simulink library "FCM_lib"  (Simulink 7.4)
settings: Solver=ode45  StartTime=0.0  StopTime=10.0  RelTol=1e-3
values from neighbouring files (symbols this model uses):
  FCMc_c_BCPNomEngy = mpt.Parameter    [FCM_CAL.m]
  FCMc_c_BRMRatCpty = mpt.Parameter    [FCM_CAL.m]
  FCMc_enum_BRMBattType = mpt.Parameter    [FCM_CAL.m]
  FCMc_i_ConstCurReq = mpt.Parameter    [FCM_CAL.m]
  FCMc_i_CurDifThrld = mpt.Parameter    [FCM_CAL.m]
  FCMc_i_CurReq_min = mpt.Parameter    [FCM_CAL.m]
  FCMc_num_BRMProtolVer = mpt.Parameter    [FCM_CAL.m]
  FCMc_t_CellTemp_MaxAlwd = mpt.Parameter    [FCM_CAL.m]
  FCMc_t_CellTemp_MinAlwd = mpt.Parameter    [FCM_CAL.m]
  FCMc_tm_ConstVoltTime = mpt.Parameter    [FCM_CAL.m]
  FCMc_tm_FastEndCondt = mpt.Parameter    [FCM_CAL.m]
  FCMc_v_BRMPackRatVolt = mpt.Parameter    [FCM_CAL.m]
  FCMc_v_VoltDifThrld = mpt.Parameter    [FCM_CAL.m]
  FCMm_c_CellChaC_AH = mpt.Parameter    [FCM_CAL.m]
  FCMm_i_CurrArrayT = mpt.Parameter    [FCM_CAL.m]
  FCMx_t_CelltempArrayT = mpt.Parameter    [FCM_CAL.m]
undefined symbols (not defined in the file or in its folder): BATc_pct_PackSocAlwd, BATc_v_CellVolt_MaxAlwd, BATc_v_CellVolt_MinAlwd, BATc_v_ConstVoltCell, BATc_v_PackVoltAlwd, FCM_Charging_St, PACK_Const_ParaCellNumOfMdl
libraries: Defined_Functionality x18
(part 1 of 2)
settings Model: Creator=sunsijun  LastModifiedBy=sunsijun

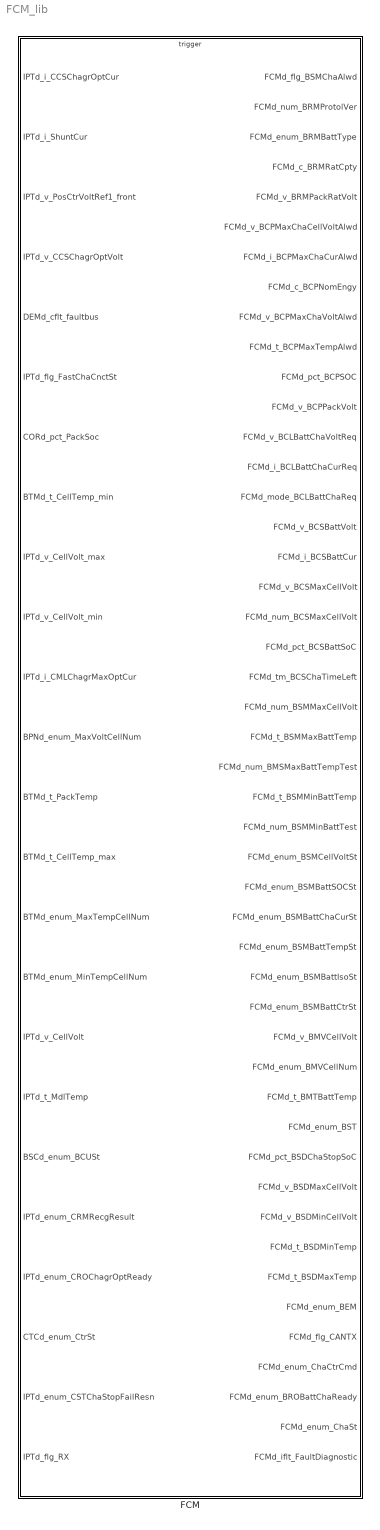
== system FCM_lib ==
  FCM : Subsystem  Description=|  TreatAsAtomicUnit=on
      | $Author:zwy
      | $Date:2015/05/12$    
      | $Revision:1.0$
      settings: RTWSystemCode=Function  RTWFcnNameOpts=Use subsystem name

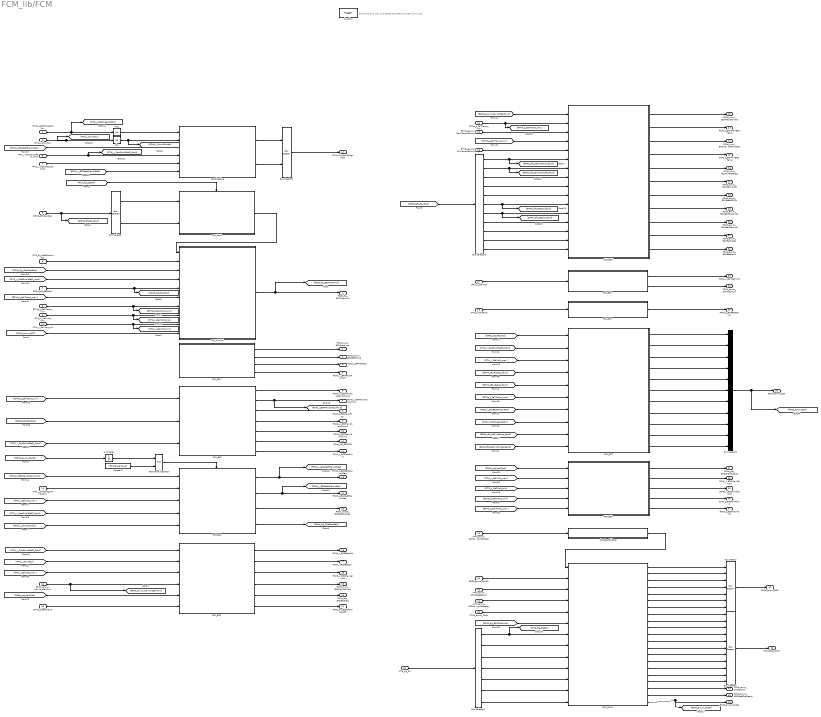
== system FCM_lib/FCM ==
  note: $Author:Zhang Weiyou$
      | $Date:2015/06/10-$
      | $Revision:1.0$
  IPTd_i_CCSChagrOptCur : Inport
  IPTd_i_ShuntCur : Inport  Port=2
  IPTd_v_PosCtrVoltRef1_front : Inport  Port=3
  IPTd_v_CCSChagrOptVolt : Inport  Port=4
  DEMd_cflt_faultbus : Inport  Port=5
  IPTd_flg_FastChaCnctSt : Inport  Port=6
  CORd_pct_PackSoc : Inport  Port=7
  BTMd_t_CellTemp_min : Inport  Port=8
  IPTd_v_CellVolt_max : Inport  Port=9
  IPTd_v_CellVolt_min : Inport  Port=10
  IPTd_i_CMLChagrMaxOptCur : Inport  Port=11
  BPNd_enum_MaxVoltCellNum : Inport  Port=12
  BTMd_t_PackTemp : Inport  Port=13
  BTMd_t_CellTemp_max : Inport  Port=14
  BTMd_enum_MaxTempCellNum : Inport  Port=15
  BTMd_enum_MinTempCellNum : Inport  Port=16
  IPTd_v_CellVolt : Inport  Port=17
  IPTd_t_MdlTemp : Inport  Port=18
  BSCd_enum_BCUSt : Inport  Port=19
  IPTd_enum_CRMRecgResult : Inport  Port=20
  IPTd_enum_CROChagrOptReady : Inport  Port=21
  CTCd_enum_CtrSt : Inport  Port=22
  IPTd_enum_CSTChaStopFailResn : Inport  Port=23
  IPTd_flg_RX : Inport  Port=24
  function : TriggerPort  TriggerType=function-call
  Abs : Abs
  Abs1 : Abs
  Bus Creator : BusCreator  Inputs=7
  Bus Creator1 : BusCreator  Inputs=11
  Bus Creator2 : BusCreator  Inputs=11
  Bus Creator3 : BusCreator  Inputs=2
  Bus Selector : BusSelector  OutputSignals=FCM_Fault_Bus.FCMd_cflt_ChaCurDifOver_faultRaw,FCM_Fault_Bus.FCMd_cflt_ChaVoltDifOver_faultRaw
  Bus Selector1 : BusSelector  OutputSignals=BPN_Fault_Bus.BPNd_cflt_CellVoltOver_faultRaw,BPN_Fault_Bus.BPNd_cflt_CellVoltUnder_faultRaw,BPN_Fault_Bus.BPNd_cflt_PackVoltUnder_faultRaw,BPN_Fault_Bus.BPNd_cflt_PackVoltOver_faultRaw,BPN_Fault_Bus.BPNd_cflt_ChaCurOver_faultRaw,EHP_Fault_Bus.EHPd_cflt_PosIso_faultRaw,EHP_Fault_Bus.EHPd_cflt_NegIso_faultRaw,CTC_Fault_Bus.CTCd_cflt_PosCtrStuckOpen_faultRaw,CTC_Fault_Bus.CTCd_cflt_PosCtrStuckCld_faultRaw,CTC_Fault_Bus.CTCd_cflt_NegCtrStuckOpen_faultRaw,CTC_Fault_Bus.CTCd_cflt_NegCtrStuckCld_faultRaw
  Bus Selector2 : BusSelector  OutputSignals=IPTd_flg_CCSRX,IPTd_flg_CMLRX,IPTd_flg_CRORX,IPTd_flg_CSDRX,IPTd_flg_CSTRX,IPTd_flg_CTSRX,IPTd_flg_CRMRX
  ChaStopFailResn : Subsystem
  Constant : Constant  Value=FCM_Charging_St  OutDataTypeMode=uint8  OutDataType=fixdt(1, 16)  OutScaling=2^0  OutDataTypeStr=uint8
  FCM_BCL : Subsystem
      settings: RTWFcnNameOpts=Use subsystem name  RTWFileNameOpts=Use subsystem name
  FCM_BCP : Subsystem
      settings: RTWFcnNameOpts=Use subsystem name  RTWFileNameOpts=Use subsystem name
  FCM_BCS : Subsystem
      settings: RTWFcnNameOpts=Use subsystem name  RTWFileNameOpts=Use subsystem name
  FCM_BMT : Subsystem
      settings: RTWFcnNameOpts=Use subsystem name  RTWFileNameOpts=Use subsystem name
  FCM_BMV : Subsystem
      settings: RTWFcnNameOpts=Use subsystem name  RTWFileNameOpts=Use subsystem name
  FCM_BRM : Subsystem
      settings: RTWFcnNameOpts=Use subsystem name  RTWFileNameOpts=Use subsystem name
  FCM_BSD : Subsystem
      settings: RTWFcnNameOpts=Use subsystem name  RTWFileNameOpts=Use subsystem name
  FCM_BSM : Subsystem
      settings: RTWFcnNameOpts=Use subsystem name  RTWFileNameOpts=Use subsystem name
  FCM_BST : Subsystem
      settings: RTWFcnNameOpts=Use subsystem name  RTWFileNameOpts=Use subsystem name
  FCM_ChAlwd : Subsystem
      settings: RTWFcnNameOpts=Use subsystem name  RTWFileNameOpts=Use subsystem name
  FCM_FLOW : Stateflow chart
      settings: RTWFcnNameOpts=Use subsystem name  RTWFileNameOpts=Use subsystem name
  FCM_fault : Subsystem  Description=|
      | $Author:Zhao XiangRi$
      | $Date:2015/03/30$    
      | $Revision:1.0$
  FastChaDiag : Subsystem  Description=|
      | $Author:Zhao XiangRi$
      | $Date:2015/03/30$    
      | $Revision:1.0$
  Relational Operator : RelationalOperator  Operator===  LogicOutDataTypeMode=boolean  LogicDataType=fixdt(0, 8)  OutDataTypeStr=boolean
  Unit Delay : UnitDelay  SampleTime=-1
  FCMd_flg_BSMChaAlwd : Outport
  FCMd_num_BRMProtolVer : Outport  Port=2
  FCMd_enum_BRMBattType : Outport  Port=3
  FCMd_c_BRMRatCpty : Outport  Port=4
  FCMd_v_BRMPackRatVolt : Outport  Port=5
  FCMd_v_BCPMaxChaCellVoltAlwd : Outport  Port=6
  FCMd_i_BCPMaxChaCurAlwd : Outport  Port=7
  FCMd_c_BCPNomEngy : Outport  Port=8
  FCMd_v_BCPMaxChaVoltAlwd : Outport  Port=9
  FCMd_t_BCPMaxTempAlwd : Outport  Port=10
  FCMd_pct_BCPSOC : Outport  Port=11
  FCMd_v_BCPPackVolt : Outport  Port=12
  FCMd_v_BCLBattChaVoltReq : Outport  Port=13
  FCMd_i_BCLBattChaCurReq : Outport  Port=14
  FCMd_mode_BCLBattChaReq : Outport  Port=15
  FCMd_v_BCSBattVolt : Outport  Port=16
  FCMd_i_BCSBattCur : Outport  Port=17
  FCMd_v_BCSMaxCellVolt : Outport  Port=18
  FCMd_num_BCSMaxCellVolt : Outport  Port=19
  FCMd_pct_BCSBattSoC : Outport  Port=20
  FCMd_tm_BCSChaTimeLeft : Outport  Port=21
  FCMd_num_BSMMaxCellVolt : Outport  Port=22
  FCMd_t_BSMMaxBattTemp : Outport  Port=23
  FCMd_num_BMSMaxBattTempTest : Outport  Port=24
  FCMd_t_BSMMinBattTemp : Outport  Port=25
  FCMd_num_BSMMinBattTest : Outport  Port=26
  FCMd_enum_BSMCellVoltSt : Outport  Port=27
  FCMd_enum_BSMBattSOCSt : Outport  Port=28
  FCMd_enum_BSMBattChaCurSt : Outport  Port=29
  FCMd_enum_BSMBattTempSt : Outport  Port=30
  FCMd_enum_BSMBattIsoSt : Outport  Port=31
  FCMd_enum_BSMBattCtrSt : Outport  Port=32
  FCMd_v_BMVCellVolt : Outport  Port=33
  FCMd_enum_BMVCellNum : Outport  Port=34  InitialOutput=0
  FCMd_t_BMTBattTemp : Outport  Port=35
  FCMd_enum_BST : Outport  Port=36
  FCMd_pct_BSDChaStopSoC : Outport  Port=37
  FCMd_v_BSDMaxCellVolt : Outport  Port=38
  FCMd_v_BSDMinCellVolt : Outport  Port=39
  FCMd_t_BSDMinTemp : Outport  Port=40
  FCMd_t_BSDMaxTemp : Outport  Port=41
  FCMd_enum_BEM : Outport  Port=42
  FCMd_flg_CANTX : Outport  Port=43
  FCMd_enum_ChaCtrCmd : Outport  Port=44
  FCMd_enum_BROBattChaReady : Outport  Port=45
  FCMd_enum_ChaSt : Outport  Port=46
  FCMd_iflt_FaultDiagnostic : Outport  Port=47
  wires:
  Relational Operator/1 -> FCM_BCL/Enable
  Unit Delay/1 -> Relational Operator/1
  Constant/1 -> Relational Operator/2
  [FCMd_enum_ChaSt] -> Unit Delay/1
  [IPTd_flg_CCSRX] -> FCM_fault/Enable
  [FCMd_enum_BST] -> FCM_ChAlwd/10(FCMd_enum_BST)
  FCM_fault/1(FCMd_flg_fault) -> FCM_ChAlwd/1(FCMd_flg_fault)
  Abs/1 -> [FCMd_i_ShuntCurAbs], FastChaDiag/2(FCMd_i_ShuntCurAbs)  "FCMd_i_ShuntCurAbs"
  Abs1/1 -> FastChaDiag/1(FCMd_i_CCSChagrOptCurAbs)  "FCMd_i_CCSChagrOptCurAbs"
  [IPTd_v_PosCtrVoltRef1_front] -> FCM_ChAlwd/4(IPTd_v_PosCtrVoltRef1_front)
  DEMd_cflt_faultbus/1 -> [DEMd_cflt_faultbus], Bus Selector/1
  Bus Creator3/1 -> FCMd_iflt_FaultDiagnostic/1  "FCMd_iflt_FaultDiagnostic"
  FastChaDiag/2(FCMd_iflt_ChaVoltDifOver_fault) -> Bus Creator3/2
  FastChaDiag/1(FCMd_iflt_ChaCurDifOver_fault) -> Bus Creator3/1
  [FCMd_v_BCLBattChaVoltReq] -> FastChaDiag/6(FCMd_v_BCLBattChaVoltReq)
  IPTd_v_CCSChagrOptVolt/1 -> FastChaDiag/5(IPTd_v_CCSChagrOptVolt)
  [FCMd_i_BCLBattChaCurReq] -> FastChaDiag/3(FCMd_i_BCLBattChaCurReq)
  IPTd_v_PosCtrVoltRef1_front/1 -> [IPTd_v_PosCtrVoltRef1_front], FastChaDiag/4(IPTd_v_PosCtrVoltRef1_front)
  IPTd_i_CCSChagrOptCur/1 -> [IPTd_i_CCSChagrOptCur], Abs1/1
  [FCMd_i_ShuntCurAbs] -> FCM_BCL/5(FCMd_i_ShuntCurAbs)
  Bus Selector2/7 -> FCM_FLOW/13(IPTd_flg_CRMRX)  "<IPTd_flg_CRMRX>"
  Bus Selector2/2 -> FCM_FLOW/8(IPTd_flg_CMLRX)  "<IPTd_flg_CMLRX>"
  Bus Selector2/6 -> FCM_FLOW/12(IPTd_flg_CTSRX)  "<IPTd_flg_CTSRX>"
  Bus Selector2/1 -> [IPTd_flg_CCSRX], FCM_FLOW/7(IPTd_flg_CCSRX)  "<IPTd_flg_CCSRX>"
  Bus Selector2/4 -> FCM_FLOW/10(IPTd_flg_CSDRX)  "<IPTd_flg_CSDRX>"
  Bus Selector2/5 -> FCM_FLOW/11(IPTd_flg_CSTRX)  "<IPTd_flg_CSTRX>"
  Bus Selector2/3 -> FCM_FLOW/9(IPTd_flg_CRORX)  "<IPTd_flg_CRORX>"
  FCM_FLOW/20(FCMd_enum_BROBattChaReady) -> FCMd_enum_BROBattChaReady/1  "FCMd_enum_BROBattChaReady"
  FCM_FLOW/19(FCMd_enum_ChaCtrCmd) -> FCMd_enum_ChaCtrCmd/1  "FCMd_enum_ChaCtrCmd"
  [DEMd_cflt_faultbus] -> Bus Selector1/1
  FCM_BCL/4(FCMd_flg_ChaStopReq) -> [FCMd_flg_ChaStopReq]
  [EHPd_cflt_POSIso_fault] -> FCM_BST/4(EHPd_cflt_POSIso_fault)
  [EHPd_cflt_NegIso_fault] -> FCM_BST/5(EHPd_cflt_NegIso_fault)
  [BTMd_t_CellTemp_max] -> FCM_BST/6(BTMd_t_CellTemp_max)
  [CORd_pct_PackSoc] -> FCM_BSD/1(CORd_pct_PackSoc)
  [BTMd_t_CellTemp_max] -> FCM_BSD/5(BTMd_t_CellTemp_max)
  [BTMd_t_CellTemp_min] -> FCM_BSD/4(BTMd_t_CellTemp_min)
  FCM_BSD/1(FCMd_pct_BSDChaStopSoC) -> FCMd_pct_BSDChaStopSoC/1
  FCM_BSD/2(FCMd_v_BSDMaxCellVolt) -> FCMd_v_BSDMaxCellVolt/1
  FCM_BSD/3(FCMd_v_BSDMinCellVolt) -> FCMd_v_BSDMinCellVolt/1
  FCM_BSD/4(FCMd_t_BSDMinTemp) -> FCMd_t_BSDMinTemp/1
  FCM_BSD/5(FCMd_t_BSDMaxTemp) -> FCMd_t_BSDMaxTemp/1
  [IPTd_v_CellVolt_max] -> FCM_BSD/2(IPTd_v_CellVolt_max)
  [IPTd_v_CellVolt_min] -> FCM_BSD/3(IPTd_v_CellVolt_min)
  [BPNd_cflt_CellVoltOver_fault] -> FCM_BST/9(BPNd_cflt_CellVoltOver_fault)
  FCM_BST/1(FCMd_enum_BSTChaStopResn1) -> Bus Creator2/1
  FCM_BST/2(FCMd_enum_BSTChaStopResn2) -> Bus Creator2/2
  FCM_BST/3(FCMd_enum_BSTChaStopResn3) -> Bus Creator2/3
  FCM_BST/4(FCMd_enum_BSTChaFailResn1) -> Bus Creator2/4
  FCM_BST/5(FCMd_enum_BSTChaFailResn2) -> Bus Creator2/5
  FCM_BST/6(FCMd_enum_BSTChaFailResn3) -> Bus Creator2/6
  FCM_BST/7(FCMd_enum_BSTChaFailResn4) -> Bus Creator2/7
  FCM_BST/8(FCMd_enum_BSTChaFailResn5) -> Bus Creator2/8
  FCM_BST/9(FCMd_enum_BSTChaFailResn6) -> Bus Creator2/9
  FCM_BST/10(FCMd_enum_BSTChaErrResn1) -> Bus Creator2/10
  FCM_BST/11(FCMd_enum_BSTChaErrResn2) -> Bus Creator2/11
  [CORd_pct_PackSoc] -> FCM_BST/1(CORd_pct_PackSoc)
  [IPTd_v_PosCtrVoltRef1_front] -> FCM_BST/2(IPTd_v_PosCtrVoltRef1_front)
  [IPTd_v_CellVolt_max] -> FCM_BST/3(IPTd_v_CellVolt_max)
  Bus Creator2/1 -> [FCMd_enum_BST], FCMd_enum_BST/1  "FCMd_enum_BST"
  FCM_BCS/1(FCMd_v_BCSBattVolt) -> FCMd_v_BCSBattVolt/1
  FCM_BCS/2(FCMd_i_BCSBattCur) -> FCMd_i_BCSBattCur/1
  FCM_BCS/3(FCMd_v_BCSMaxCellVolt) -> FCMd_v_BCSMaxCellVolt/1
  FCM_BCS/4(FCMd_num_BCSMaxCellVolt) -> FCMd_num_BCSMaxCellVolt/1
  FCM_BCS/5(FCMd_pct_BCSBattSoC) -> FCMd_pct_BCSBattSoC/1
  [IPTd_v_PosCtrVoltRef1_front] -> FCM_BCS/1("IPTd_v_PosCtrVoltRef1_front ")
  BPNd_enum_MaxVoltCellNum/1 -> [BPNd_enum_MaxVoltCellNum], FCM_BCS/4(BPNd_enum_MaxVoltCellNum)
  [IPTd_v_CellVolt_max] -> FCM_BCS/3(IPTd_v_CellVolt_max)
  [CORd_pct_PackSoc] -> FCM_BCS/5(CORd_pct_PackSoc)
  BTMd_t_PackTemp/1 -> FCM_BCS/6(BTMd_t_PackTemp)
  FCM_BCS/6(FCMd_tm_BCSChaTimeLeft) -> FCMd_tm_BCSChaTimeLeft/1
  [IPTd_i_ShuntCur] -> FCM_BCS/2(IPTd_i_ShuntCur)
  Bus Selector1/1 -> FCM_BSM/6(BPNd_cflt_CellVoltOver_fault), [BPNd_cflt_CellVoltOver_fault]  "<BPNd_cflt_CellVoltOver_faultRaw>"
  Bus Selector1/2 -> FCM_BSM/7(BPNd_cflt_CellVoltUnder_fault), [BPNd_cflt_CellVoltUnder_fault]  "<BPNd_cflt_CellVoltUnder_faultRaw>"
  Bus Selector1/3 -> FCM_BSM/8(BPNd_cflt_PackSocUnder_fault)  "<BPNd_cflt_PackVoltUnder_faultRaw>"
  Bus Selector1/4 -> FCM_BSM/9(BPNd_cflt_PackSocOver_fault)  "<BPNd_cflt_PackVoltOver_faultRaw>"
  BTMd_t_CellTemp_max/1 -> FCM_BSM/2(BTMd_t_CellTemp_max), [BTMd_t_CellTemp_max]
  [BPNd_enum_MaxVoltCellNum] -> FCM_BSM/1(BPNd_enum_MaxVoltCellNum)
  BTMd_enum_MaxTempCellNum/1 -> FCM_BSM/3(BTMd_enum_MaxTempCellNum)
  [BTMd_t_CellTemp_min] -> FCM_BSM/4(BTMd_t_CellTemp_min)
  BTMd_enum_MinTempCellNum/1 -> FCM_BSM/5(BTMd_enum_MinTempCellNum)
  Bus Selector1/5 -> FCM_BSM/10(BPNd_cflt_ChaCurOver_fault)  "<BPNd_cflt_ChaCurOver_faultRaw>"
  Bus Selector1/6 -> FCM_BSM/11(EHPd_cflt_POSIso_fault), [EHPd_cflt_POSIso_fault]  "<EHPd_cflt_PosIso_faultRaw>"
  Bus Selector1/7 -> FCM_BSM/12(EHPd_cflt_NegIso_fault), [EHPd_cflt_NegIso_fault]  "<EHPd_cflt_NegIso_faultRaw>"
  Bus Selector1/8 -> FCM_BSM/13(CTCd_cflt_PosCtrStuckOpen_fault)  "<CTCd_cflt_PosCtrStuckOpen_faultRaw>"
  Bus Selector1/9 -> FCM_BSM/14(CTCd_cflt_PosCtrStuckCld_fault)  "<CTCd_cflt_PosCtrStuckCld_faultRaw>"
  Bus Selector1/10 -> FCM_BSM/15(CTCd_cflt_NegCtrtStuckOpen_fault)  "<CTCd_cflt_NegCtrStuckOpen_faultRaw>"
  Bus Selector1/11 -> FCM_BSM/16(CTCd_cflt_NegCtrStuckCld_fault)  "<CTCd_cflt_NegCtrStuckCld_faultRaw>"
  FCM_BSM/6(FCMd_enum_BSMCellVoltSt) -> FCMd_enum_BSMCellVoltSt/1
  FCM_BSM/7(FCMd_enum_BSMBattSOCSt) -> FCMd_enum_BSMBattSOCSt/1
  FCM_BSM/8(FCMd_enum_BSMBattChaCurSt) -> FCMd_enum_BSMBattChaCurSt/1
  FCM_BSM/9(FCMd_enum_BSMBattTempSt) -> FCMd_enum_BSMBattTempSt/1
  FCM_BSM/10(FCMd_enum_BSMBattIsoSt) -> FCMd_enum_BSMBattIsoSt/1
  FCM_BSM/11(FCMd_enum_BSMBattCtrSt) -> FCMd_enum_BSMBattCtrSt/1
  FCM_BSM/1(FCMd_num_BSMMaxCellVolt) -> FCMd_num_BSMMaxCellVolt/1
  FCM_BSM/2(FCMd_t_BSMMaxBattTemp) -> FCMd_t_BSMMaxBattTemp/1
  FCM_BSM/3(FCMd_num_BMSMaxBattTempTest) -> FCMd_num_BMSMaxBattTempTest/1
  FCM_BSM/4(FCMd_t_BSMMinBattTemp) -> FCMd_t_BSMMinBattTemp/1
  FCM_BSM/5(FCMd_num_BSMMinBattTest) -> FCMd_num_BSMMinBattTest/1
  IPTd_i_CMLChagrMaxOptCur/1 -> FCM_BCL/2(IPTd_i_CMLChagrMaxOptCur)
  [FCMd_i_BCPMaxChaCurAlwd] -> FCM_BCL/1(FCMd_i_BCPMaxChaCurAlwd)
  [IPTd_v_PosCtrVoltRef1_front] -> FCM_BCL/4(IPTd_v_PosCtrVoltRef1_front)
  IPTd_i_ShuntCur/1 -> [IPTd_i_ShuntCur], Abs/1
  [IPTd_v_CellVolt_max] -> FCM_BCL/3(IPTd_v_CellVolt_max)
  [IPTd_v_PosCtrVoltRef1_front] -> FCM_BCP/3(IPTd_v_PosCtrVoltRef1_front)
  [CORd_pct_PackSoc] -> FCM_BCP/2(CORd_pct_PackSoc)
  FCM_BCP/7(FCMd_v_BCPPackVolt) -> FCMd_v_BCPPackVolt/1
  FCM_BCP/6(FCMd_pct_BCPSOC) -> FCMd_pct_BCPSOC/1
  FCM_BCP/5(FCMd_t_BCPMaxTempAlwd) -> FCMd_t_BCPMaxTempAlwd/1
  FCM_BCP/3(FCMd_c_BCPNomEngy) -> FCMd_c_BCPNomEngy/1
  [BTMd_t_CellTemp_min] -> FCM_BCP/1(BTMd_t_CellTemp_min)
  FCM_BCP/2(FCMd_i_BCPMaxChaCurAlwd) -> [FCMd_i_BCPMaxChaCurAlwd], FCMd_i_BCPMaxChaCurAlwd/1
  FCM_BCP/1(FCMd_v_BCPMaxChaCellVoltAlwd) -> FCMd_v_BCPMaxChaCellVoltAlwd/1
  FCM_BCP/4(FCMd_v_BCPMaxChaVoltAlwd) -> FCMd_v_BCPMaxChaVoltAlwd/1
  FCM_BRM/3(FCMd_c_BRMRatCpty) -> FCMd_c_BRMRatCpty/1
  FCM_BRM/4(FCMd_v_BRMPackRatVolt) -> FCMd_v_BRMPackRatVolt/1
  IPTd_v_CellVolt/1 -> FCM_BMV/1(IPTd_v_CellVolt)
  FCM_BMV/2(FCMd_enum_BMVCellNum) -> FCMd_enum_BMVCellNum/1
  FCM_BMV/1(FCMd_v_BMVCellVolt) -> FCMd_v_BMVCellVolt/1
  IPTd_t_MdlTemp/1 -> FCM_BMT/1(IPTd_t_MdlTemp)
  FCM_BMT/1(FCMd_t_BMTBattTemp) -> FCMd_t_BMTBattTemp/1
  IPTd_flg_FastChaCnctSt/1 -> FCM_ChAlwd/2(IPTd_flg_FastChaCnctSt)
  IPTd_v_CellVolt_max/1 -> [IPTd_v_CellVolt_max], FCM_ChAlwd/8(IPTd_v_CellVolt_max)
  CORd_pct_PackSoc/1 -> [CORd_pct_PackSoc], FCM_ChAlwd/5(CORd_pct_PackSoc)
  Bus Creator/1 -> FCMd_enum_BEM/1  "FCMd_enum_BEM"
  Bus Creator1/1 -> FCMd_flg_CANTX/1  "FCMd_flg_CANTX"
  Bus Selector/1 -> FCM_fault/1(FCMd_cflt_ChaCurDifOver_fault)  "<FCMd_cflt_ChaCurDifOver_faultRaw>"
  Bus Selector/2 -> FCM_fault/2(FCMd_cflt_ChaVoltDifOver_fault)  "<FCMd_cflt_ChaVoltDifOver_faultRaw>"
  FCM_ChAlwd/1(FCMd_flg_BSMChaAlwd) -> FCMd_flg_BSMChaAlwd/1, [FCMd_flg_BSMChaAlwd]
  [FCMd_flg_ChaStopReq] -> FCM_ChAlwd/3(FCMd_flg_ChaStopReq)
  [BTMd_t_CellTemp_max] -> FCM_ChAlwd/6(BTMd_t_CellTemp_max)
  IPTd_v_CellVolt_min/1 -> FCM_ChAlwd/9(IPTd_v_CellVolt_min), [IPTd_v_CellVolt_min]
  BTMd_t_CellTemp_min/1 -> FCM_ChAlwd/7(BTMd_t_CellTemp_min), [BTMd_t_CellTemp_min]
  [IPTd_i_CCSChagrOptCur] -> FCM_BST/8(IPTd_i_CCSChagrOptCur)
  [FCMd_i_BCLBattChaCurReq] -> FCM_BST/7(FCMd_i_BCLBattChaCurReq)
  [BPNd_cflt_CellVoltUnder_fault] -> FCM_BST/10(BPNd_cflt_CellVoltUnder_fault)
  FCM_FLOW/1(FCMd_enum_BEMTimeOver3901) -> Bus Creator/1  "FCMd_enum_BEMTimeOver3901"
  FCM_FLOW/2(FCMd_enum_BEMTimeOver3902) -> Bus Creator/2  "FCMd_enum_BEMTimeOver3902"
  FCM_FLOW/3(FCMd_enum_BEMTimeOver3903) -> Bus Creator/3  "FCMd_enum_BEMTimeOver3903"
  FCM_FLOW/4(FCMd_enum_BEMTimeOver3904) -> Bus Creator/4  "FCMd_enum_BEMTimeOver3904"
  FCM_FLOW/5(FCMd_enum_BEMTimeOver3905) -> Bus Creator/5  "FCMd_enum_BEMTimeOver3905"
  FCM_FLOW/6(FCMd_enum_BEMTimeOver3906) -> Bus Creator/6  "FCMd_enum_BEMTimeOver3906"
  FCM_FLOW/7(FCMd_enum_BEMTimeOver3907) -> Bus Creator/7  "FCMd_enum_BEMTimeOver3907"
  FCM_FLOW/8(FCMd_flg_BRMTM) -> Bus Creator1/1  "FCMd_flg_BRMTM"
  FCM_FLOW/9(FCMd_flg_BCPTM) -> Bus Creator1/2  "FCMd_flg_BCPTM"
  FCM_FLOW/10(FCMd_flg_BROTM) -> Bus Creator1/3  "FCMd_flg_BROTM"
  FCM_FLOW/11(FCMd_flg_BCLTM) -> Bus Creator1/4  "FCMd_flg_BCLTM"
  FCM_FLOW/12(FCMd_flg_BCSTM) -> Bus Creator1/5  "FCMd_flg_BCSTM"
  FCM_FLOW/13(FCMd_flg_BSMTM) -> Bus Creator1/6  "FCMd_flg_BSMTM"
  FCM_FLOW/14(FCMd_flg_BMVTM) -> Bus Creator1/7  "FCMd_flg_BMVTM"
  FCM_FLOW/15(FCMd_flg_BMTTM) -> Bus Creator1/8  "FCMd_flg_BMTTM"
  FCM_FLOW/16(FCMd_flg_BSTTM) -> Bus Creator1/9  "FCMd_flg_BSTTM"
  FCM_FLOW/17(FCMd_flg_BSDTM) -> Bus Creator1/10  "FCMd_flg_BSDTM"
  FCM_FLOW/18(FCMd_flg_BEMTM) -> Bus Creator1/11  "FCMd_flg_BEMTM"
  FCM_BCL/1(FCMd_v_BCLBattChaVoltReq) -> FCMd_v_BCLBattChaVoltReq/1, [FCMd_v_BCLBattChaVoltReq]
  FCM_BCL/2(FCMd_i_BCLBattChaCurReq) -> [FCMd_i_BCLBattChaCurReq], FCMd_i_BCLBattChaCurReq/1
  FCM_BCL/3(FCMd_mode_BCLBattChaReq) -> FCMd_mode_BCLBattChaReq/1
  IPTd_enum_CRMRecgResult/1 -> FCM_FLOW/3(IPTd_enum_CRMRecgResult)
  IPTd_enum_CROChagrOptReady/1 -> FCM_FLOW/4(IPTd_enum_CROChagrOptReady)
  [FCMd_flg_BSMChaAlwd] -> FCM_FLOW/6(FCMd_flg_BSMChaAlwd)
  FCM_FLOW/21(FCMd_enum_ChaSt) -> [FCMd_enum_ChaSt], FCMd_enum_ChaSt/1  "FCMd_enum_ChaSt"
  BSCd_enum_BCUSt/1 -> FCM_FLOW/2(BSCd_enum_BCUSt)
  FCM_BRM/1(FCMd_num_BRMProtolVer) -> FCMd_num_BRMProtolVer/1
  FCM_BRM/2(FCMd_enum_BRMBattType) -> FCMd_enum_BRMBattType/1
  CTCd_enum_CtrSt/1 -> FCM_FLOW/5(CTCd_enum_CtrSt)
  IPTd_enum_CSTChaStopFailResn/1 -> ChaStopFailResn/1(IPTd_enum_CSTChaStopFailResn)
  ChaStopFailResn/1(FCMd_flg_CSTChaStop) -> FCM_FLOW/1(FCMd_flg_CSTChaStop)
  IPTd_flg_RX/1 -> Bus Selector2/1

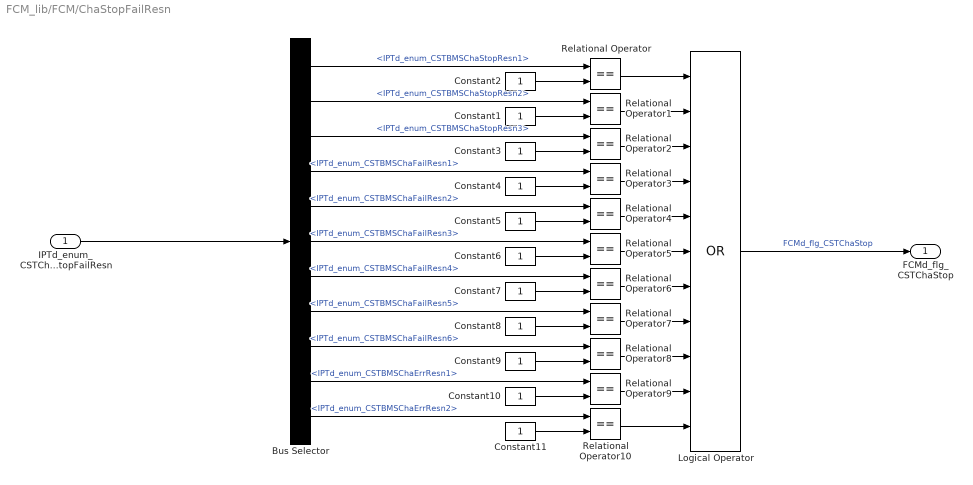
== system FCM_lib/FCM/ChaStopFailResn ==
  IPTd_enum_CSTChaStopFailResn : Inport
  Bus Selector : BusSelector  OutputSignals=IPTd_enum_CSTBMSChaStopResn1,IPTd_enum_CSTBMSChaStopResn2,IPTd_enum_CSTBMSChaStopResn3,IPTd_enum_CSTBMSChaFailResn1,IPTd_enum_CSTBMSChaFailResn2,IPTd_enum_CSTBMSChaFailResn3,IPTd_enum_CSTBMSChaFailResn4,IPTd_enum_CSTBMSChaFailResn5,IPTd_enum_CSTBMSChaFailResn6,IPTd_enum_CSTBMSChaErrResn1,IPTd_enum_CSTBMSChaErrResn2
  Constant{1..11} (11 alike) : Constant  OutDataTypeMode=uint8  OutDataTypeStr=uint8
  Logical Operator : Logic  Operator=OR  Inputs=11  AllPortsSameDT=off
  Relational Operator{,1..10} (11 alike) : RelationalOperator  Operator===  LogicOutDataTypeMode=boolean  LogicDataType=fixdt(0, 8)  OutDataTypeStr=boolean
  FCMd_flg_CSTChaStop : Outport
  wires:
  IPTd_enum_CSTChaStopFailResn/1 -> Bus Selector/1
  Constant2/1 -> Relational Operator/2
  Logical Operator/1 -> FCMd_flg_CSTChaStop/1  "FCMd_flg_CSTChaStop"
  Relational Operator/1 -> Logical Operator/1
  Bus Selector/1 -> Relational Operator/1  "<IPTd_enum_CSTBMSChaStopResn1>"
  Constant1/1 -> Relational Operator1/2
  Bus Selector/2 -> Relational Operator1/1  "<IPTd_enum_CSTBMSChaStopResn2>"
  Constant3/1 -> Relational Operator2/2
  Constant4/1 -> Relational Operator3/2
  Constant5/1 -> Relational Operator4/2
  Constant6/1 -> Relational Operator5/2
  Constant7/1 -> Relational Operator6/2
  Constant8/1 -> Relational Operator7/2
  Constant9/1 -> Relational Operator8/2
  Constant10/1 -> Relational Operator9/2
  Relational Operator1/1 -> Logical Operator/2
  Relational Operator2/1 -> Logical Operator/3
  Relational Operator3/1 -> Logical Operator/4
  Relational Operator4/1 -> Logical Operator/5
  Relational Operator5/1 -> Logical Operator/6
  Relational Operator6/1 -> Logical Operator/7
  Relational Operator7/1 -> Logical Operator/8
  Relational Operator8/1 -> Logical Operator/9
  Relational Operator9/1 -> Logical Operator/10
  Constant11/1 -> Relational Operator10/2
  Relational Operator10/1 -> Logical Operator/11
  Bus Selector/3 -> Relational Operator2/1  "<IPTd_enum_CSTBMSChaStopResn3>"
  Bus Selector/4 -> Relational Operator3/1  "<IPTd_enum_CSTBMSChaFailResn1>"
  Bus Selector/5 -> Relational Operator4/1  "<IPTd_enum_CSTBMSChaFailResn2>"
  Bus Selector/6 -> Relational Operator5/1  "<IPTd_enum_CSTBMSChaFailResn3>"
  Bus Selector/7 -> Relational Operator6/1  "<IPTd_enum_CSTBMSChaFailResn4>"
  Bus Selector/8 -> Relational Operator7/1  "<IPTd_enum_CSTBMSChaFailResn5>"
  Bus Selector/9 -> Relational Operator8/1  "<IPTd_enum_CSTBMSChaFailResn6>"
  Bus Selector/10 -> Relational Operator9/1  "<IPTd_enum_CSTBMSChaErrResn1>"
  Bus Selector/11 -> Relational Operator10/1  "<IPTd_enum_CSTBMSChaErrResn2>"

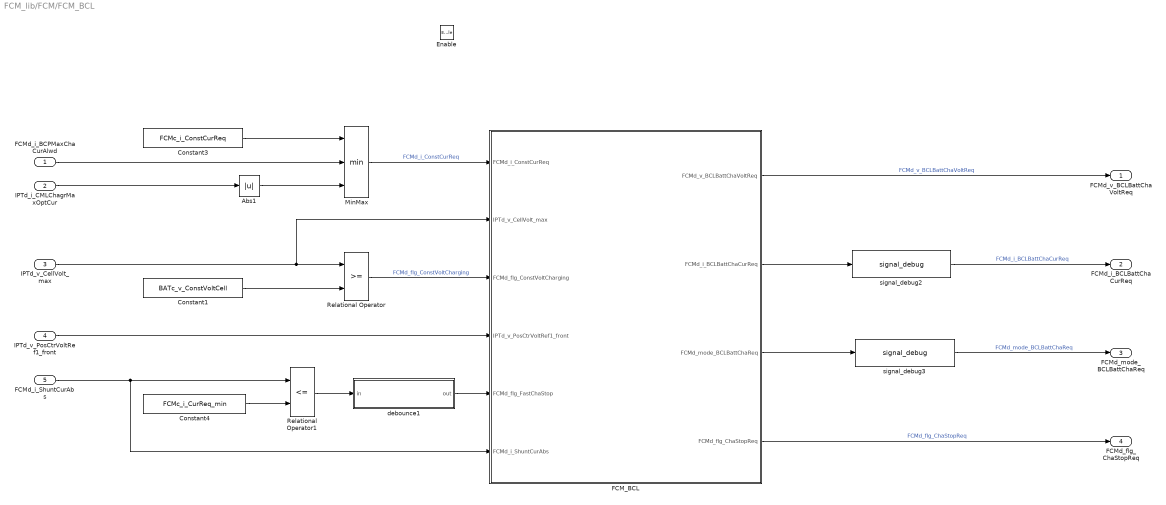
== system FCM_lib/FCM/FCM_BCL ==
  FCMd_i_BCPMaxChaCurAlwd : Inport
  IPTd_i_CMLChagrMaxOptCur : Inport  Port=2
  IPTd_v_CellVolt_max : Inport  Port=3
  IPTd_v_PosCtrVoltRef1_front : Inport  Port=4
  FCMd_i_ShuntCurAbs : Inport  Port=5
  Enable : EnablePort
  Abs1 : Abs
  Constant1 : Constant  Value=BATc_v_ConstVoltCell
  Constant3 : Constant  Value=FCMc_i_ConstCurReq
  Constant4 : Constant  Value=FCMc_i_CurReq_min
  FCM_BCL : Stateflow chart  TreatAsAtomicUnit=on
  MinMax : MinMax  Inputs=3
  Relational Operator : RelationalOperator  LogicOutDataTypeMode=boolean  LogicDataType=fixdt(0, 8)  OutDataTypeStr=boolean
  Relational Operator1 : RelationalOperator  Operator=<=  LogicOutDataTypeMode=boolean  LogicDataType=fixdt(0, 8)  OutDataTypeStr=boolean
  debounce1 : Subsystem  TreatAsAtomicUnit=on  RTWFcnName=debounce1  mask(debounce){debounce_time=FCMc_tm_FastEndCondt}
      mask prompts: debounce_time "debounce_time_ms"
      mask help: Debounce the input digital signal.
      settings: AttributesFormatString=[DEBOUNCE_TIME=%<debounce_time>]  RTWFcnNameOpts=User specified
      mask Display:
      | disp('DEBOUNCE')
      | port_label('input',1,'in')
      | port_label('output',1,'out')
  signal_debug2 : Defined_Functionality/signal_debug  SystemSampleTime=-1  debug_switch=FCMc_dbgsw_BCLBattChaCurReq  debug_value=FCMc_dbgval_BCLBattChaCurReq
      settings: AttributesFormatString=[SWITCH=%<debug_switch>]\n[VALUE=%<debug_value>]
  signal_debug3 : Defined_Functionality/signal_debug  SystemSampleTime=-1  debug_switch=FCMc_dbgsw_BCLBattChaReqmode  debug_value=FCMc_dbgval_BCLBattChaReqmode
      settings: AttributesFormatString=[SWITCH=%<debug_switch>]\n[VALUE=%<debug_value>]
  FCMd_v_BCLBattChaVoltReq : Outport
  FCMd_i_BCLBattChaCurReq : Outport  Port=2
  FCMd_mode_BCLBattChaReq : Outport  Port=3
  FCMd_flg_ChaStopReq : Outport  Port=4
  wires:
  FCM_BCL/2(FCMd_i_BCLBattChaCurReq) -> signal_debug2/1
  debounce1/1(out) -> FCM_BCL/5(FCMd_flg_FastChaStop)
  Constant4/1 -> Relational Operator1/2
  Relational Operator1/1 -> debounce1/1(in)
  FCMd_i_ShuntCurAbs/1 -> FCM_BCL/6(FCMd_i_ShuntCurAbs), Relational Operator1/1
  FCM_BCL/1(FCMd_v_BCLBattChaVoltReq) -> FCMd_v_BCLBattChaVoltReq/1  "FCMd_v_BCLBattChaVoltReq"
  IPTd_v_PosCtrVoltRef1_front/1 -> FCM_BCL/4(IPTd_v_PosCtrVoltRef1_front)
  Relational Operator/1 -> FCM_BCL/3(FCMd_flg_ConstVoltCharging)  "FCMd_flg_ConstVoltCharging"
  FCM_BCL/3(FCMd_mode_BCLBattChaReq) -> signal_debug3/1
  Constant1/1 -> Relational Operator/2
  Abs1/1 -> MinMax/3
  Constant3/1 -> MinMax/1
  IPTd_v_CellVolt_max/1 -> FCM_BCL/2(IPTd_v_CellVolt_max), Relational Operator/1
  MinMax/1 -> FCM_BCL/1(FCMd_i_ConstCurReq)  "FCMd_i_ConstCurReq"
  FCMd_i_BCPMaxChaCurAlwd/1 -> MinMax/2
  signal_debug3/1 -> FCMd_mode_BCLBattChaReq/1  "FCMd_mode_BCLBattChaReq"
  IPTd_i_CMLChagrMaxOptCur/1 -> Abs1/1
  signal_debug2/1 -> FCMd_i_BCLBattChaCurReq/1  "FCMd_i_BCLBattChaCurReq"
  FCM_BCL/4(FCMd_flg_ChaStopReq) -> FCMd_flg_ChaStopReq/1  "FCMd_flg_ChaStopReq"

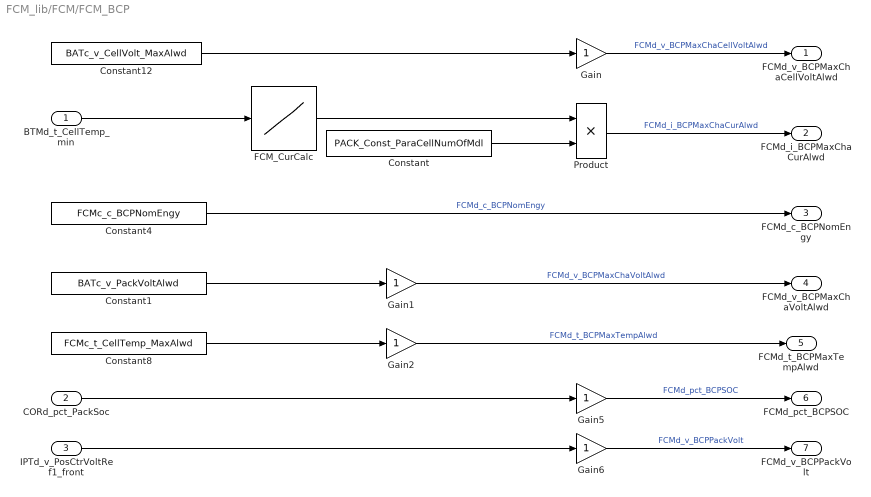
== system FCM_lib/FCM/FCM_BCP ==
  BTMd_t_CellTemp_min : Inport
  CORd_pct_PackSoc : Inport  Port=2
  IPTd_v_PosCtrVoltRef1_front : Inport  Port=3
  Constant : Constant  Value=PACK_Const_ParaCellNumOfMdl  OutDataTypeMode=uint8  OutDataTypeStr=uint8
  Constant1 : Constant  Value=BATc_v_PackVoltAlwd
  Constant12 : Constant  Value=BATc_v_CellVolt_MaxAlwd
  Constant4 : Constant  Value=FCMc_c_BCPNomEngy
  Constant8 : Constant  Value=FCMc_t_CellTemp_MaxAlwd
  FCM_CurCalc : Lookup  InputValues=FCMx_t_CelltempArrayT  Table=FCMm_i_CurrArrayT  LookUpMeth=Interpolation-Use End Values  OutDataTypeStr=Inherit: Inherit via back propagation
  Gain{,1..2,5..6} (5 alike) : Gain  OutDataTypeStr=Inherit: Inherit via back propagation
  Product : Product  OutDataTypeStr=Inherit: Same as first input
  FCMd_v_BCPMaxChaCellVoltAlwd : Outport
  FCMd_i_BCPMaxChaCurAlwd : Outport  Port=2
  FCMd_c_BCPNomEngy : Outport  Port=3
  FCMd_v_BCPMaxChaVoltAlwd : Outport  Port=4
  FCMd_t_BCPMaxTempAlwd : Outport  Port=5
  FCMd_pct_BCPSOC : Outport  Port=6
  FCMd_v_BCPPackVolt : Outport  Port=7
  wires:
  Gain2/1 -> FCMd_t_BCPMaxTempAlwd/1  "FCMd_t_BCPMaxTempAlwd"
  Constant8/1 -> Gain2/1
  Gain1/1 -> FCMd_v_BCPMaxChaVoltAlwd/1  "FCMd_v_BCPMaxChaVoltAlwd"
  Constant4/1 -> FCMd_c_BCPNomEngy/1  "FCMd_c_BCPNomEngy"
  CORd_pct_PackSoc/1 -> Gain5/1
  Gain5/1 -> FCMd_pct_BCPSOC/1  "FCMd_pct_BCPSOC"
  IPTd_v_PosCtrVoltRef1_front/1 -> Gain6/1
  Gain6/1 -> FCMd_v_BCPPackVolt/1  "FCMd_v_BCPPackVolt"
  Constant/1 -> Product/2
  Product/1 -> FCMd_i_BCPMaxChaCurAlwd/1  "FCMd_i_BCPMaxChaCurAlwd"
  BTMd_t_CellTemp_min/1 -> FCM_CurCalc/1
  FCM_CurCalc/1 -> Product/1
  Constant12/1 -> Gain/1
  Constant1/1 -> Gain1/1
  Gain/1 -> FCMd_v_BCPMaxChaCellVoltAlwd/1  "FCMd_v_BCPMaxChaCellVoltAlwd"

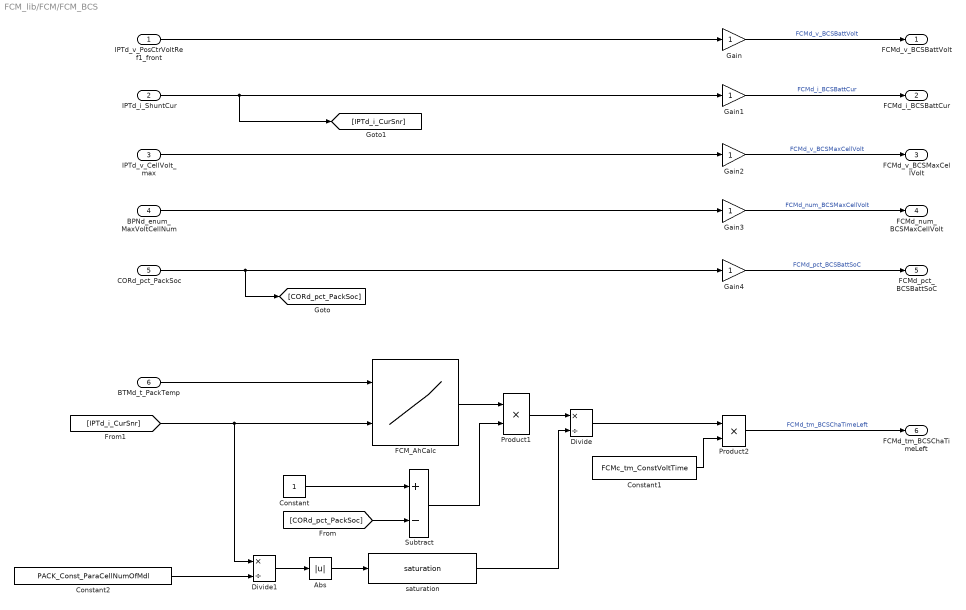
== system FCM_lib/FCM/FCM_BCS ==
  "IPTd_v_PosCtrVoltRef1_front " : Inport
  IPTd_i_ShuntCur : Inport  Port=2
  IPTd_v_CellVolt_max : Inport  Port=3
  BPNd_enum_MaxVoltCellNum : Inport  Port=4
  CORd_pct_PackSoc : Inport  Port=5
  BTMd_t_PackTemp : Inport  Port=6
  Abs : Abs  OutDataType=fixdt(1, 16)  OutScaling=2^0
  Constant : Constant  OutDataTypeMode=single  OutDataTypeStr=single
  Constant1 : Constant  Value=FCMc_tm_ConstVoltTime  OutDataTypeMode=uint8  OutDataTypeStr=uint8
  Constant2 : Constant  Value=PACK_Const_ParaCellNumOfMdl  OutDataTypeMode=single  OutDataTypeStr=single
  Divide : Product  Inputs=*/
  Divide1 : Product  Inputs=*/
  FCM_AhCalc : Lookup2D  RowIndex=FCMx_t_CellChaTemp  ColumnIndex=FCMy_i_CellChaCur  Table=FCMm_c_CellChaC_AH  LookUpMeth=Interpolation-Use End Values
  Gain{,1..4} (5 alike) : Gain  OutDataTypeStr=Inherit: Inherit via back propagation
  Product1 : Product
  Product2 : Product  OutDataTypeStr=Inherit: Inherit via back propagation
  Subtract : Sum  Inputs=+-
  saturation : Defined_Functionality/saturation  SystemSampleTime=-1  upper_limit=400  lower_limit=1
      settings: AttributesFormatString=[UPPER_LIMIT=%<upper_limit>]\n[LOWER_LIMIT=%<lower_limit>]
  FCMd_v_BCSBattVolt : Outport
  FCMd_i_BCSBattCur : Outport  Port=2
  FCMd_v_BCSMaxCellVolt : Outport  Port=3
  FCMd_num_BCSMaxCellVolt : Outport  Port=4
  FCMd_pct_BCSBattSoC : Outport  Port=5
  FCMd_tm_BCSChaTimeLeft : Outport  Port=6
  wires:
  Constant2/1 -> Divide1/2
  Divide1/1 -> Abs/1
  "IPTd_v_PosCtrVoltRef1_front "/1 -> Gain/1
  Gain/1 -> FCMd_v_BCSBattVolt/1  "FCMd_v_BCSBattVolt"
  IPTd_i_ShuntCur/1 -> Gain1/1, [IPTd_i_CurSnr]
  Gain1/1 -> FCMd_i_BCSBattCur/1  "FCMd_i_BCSBattCur"
  IPTd_v_CellVolt_max/1 -> Gain2/1
  Gain2/1 -> FCMd_v_BCSMaxCellVolt/1  "FCMd_v_BCSMaxCellVolt"
  Gain3/1 -> FCMd_num_BCSMaxCellVolt/1  "FCMd_num_BCSMaxCellVolt"
  BPNd_enum_MaxVoltCellNum/1 -> Gain3/1
  CORd_pct_PackSoc/1 -> Gain4/1, [CORd_pct_PackSoc]
  Gain4/1 -> FCMd_pct_BCSBattSoC/1  "FCMd_pct_BCSBattSoC"
  Constant/1 -> Subtract/1
  Subtract/1 -> Product1/2
  Constant1/1 -> Product2/2
  Product2/1 -> FCMd_tm_BCSChaTimeLeft/1  "FCMd_tm_BCSChaTimeLeft"
  Product1/1 -> Divide/1
  BTMd_t_PackTemp/1 -> FCM_AhCalc/1
  Divide/1 -> Product2/1
  [IPTd_i_CurSnr] -> Divide1/1, FCM_AhCalc/2
  FCM_AhCalc/1 -> Product1/1
  saturation/1 -> Divide/2
  [CORd_pct_PackSoc] -> Subtract/2
  Abs/1 -> saturation/1

== system FCM_lib/FCM/FCM_BMT ==
  IPTd_t_MdlTemp : Inport
  Gain : Gain
  FCMd_t_BMTBattTemp : Outport
  wires:
  Gain/1 -> FCMd_t_BMTBattTemp/1  "FCMd_t_BMTBattTemp"
  IPTd_t_MdlTemp/1 -> Gain/1

== system FCM_lib/FCM/FCM_BMV ==
  IPTd_v_CellVolt : Inport
  Constant2 : Constant  OutDataTypeMode=uint8  OutDataTypeStr=uint8
  Gain : Gain  OutDataTypeStr=Inherit: Inherit via back propagation
  FCMd_v_BMVCellVolt : Outport
  FCMd_enum_BMVCellNum : Outport  Port=2
  wires:
  Gain/1 -> FCMd_v_BMVCellVolt/1  "FCMd_v_BMVCellVolt"
  IPTd_v_CellVolt/1 -> Gain/1
  Constant2/1 -> FCMd_enum_BMVCellNum/1  "FCMd_enum_BMVCellNum"

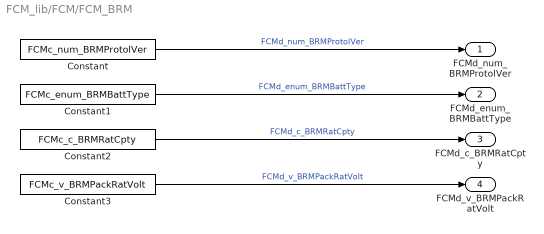
== system FCM_lib/FCM/FCM_BRM ==
  Constant : Constant  Value=FCMc_num_BRMProtolVer
  Constant1 : Constant  Value=FCMc_enum_BRMBattType
  Constant2 : Constant  Value=FCMc_c_BRMRatCpty
  Constant3 : Constant  Value=FCMc_v_BRMPackRatVolt
  FCMd_num_BRMProtolVer : Outport
  FCMd_enum_BRMBattType : Outport  Port=2
  FCMd_c_BRMRatCpty : Outport  Port=3
  FCMd_v_BRMPackRatVolt : Outport  Port=4
  wires:
  Constant/1 -> FCMd_num_BRMProtolVer/1  "FCMd_num_BRMProtolVer"
  Constant1/1 -> FCMd_enum_BRMBattType/1  "FCMd_enum_BRMBattType"
  Constant2/1 -> FCMd_c_BRMRatCpty/1  "FCMd_c_BRMRatCpty"
  Constant3/1 -> FCMd_v_BRMPackRatVolt/1  "FCMd_v_BRMPackRatVolt"

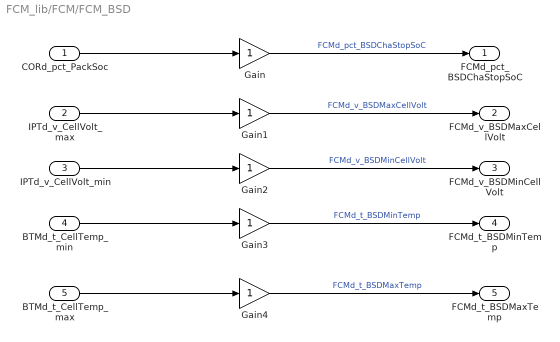
== system FCM_lib/FCM/FCM_BSD ==
  CORd_pct_PackSoc : Inport
  IPTd_v_CellVolt_max : Inport  Port=2
  IPTd_v_CellVolt_min : Inport  Port=3
  BTMd_t_CellTemp_min : Inport  Port=4
  BTMd_t_CellTemp_max : Inport  Port=5
  Gain{,1..4} (5 alike) : Gain  OutDataTypeStr=Inherit: Inherit via back propagation
  FCMd_pct_BSDChaStopSoC : Outport
  FCMd_v_BSDMaxCellVolt : Outport  Port=2
  FCMd_v_BSDMinCellVolt : Outport  Port=3
  FCMd_t_BSDMinTemp : Outport  Port=4
  FCMd_t_BSDMaxTemp : Outport  Port=5
  wires:
  IPTd_v_CellVolt_max/1 -> Gain1/1
  IPTd_v_CellVolt_min/1 -> Gain2/1
  BTMd_t_CellTemp_min/1 -> Gain3/1
  BTMd_t_CellTemp_max/1 -> Gain4/1
  CORd_pct_PackSoc/1 -> Gain/1
  Gain/1 -> FCMd_pct_BSDChaStopSoC/1  "FCMd_pct_BSDChaStopSoC"
  Gain1/1 -> FCMd_v_BSDMaxCellVolt/1  "FCMd_v_BSDMaxCellVolt"
  Gain2/1 -> FCMd_v_BSDMinCellVolt/1  "FCMd_v_BSDMinCellVolt"
  Gain4/1 -> FCMd_t_BSDMaxTemp/1  "FCMd_t_BSDMaxTemp"
  Gain3/1 -> FCMd_t_BSDMinTemp/1  "FCMd_t_BSDMinTemp"

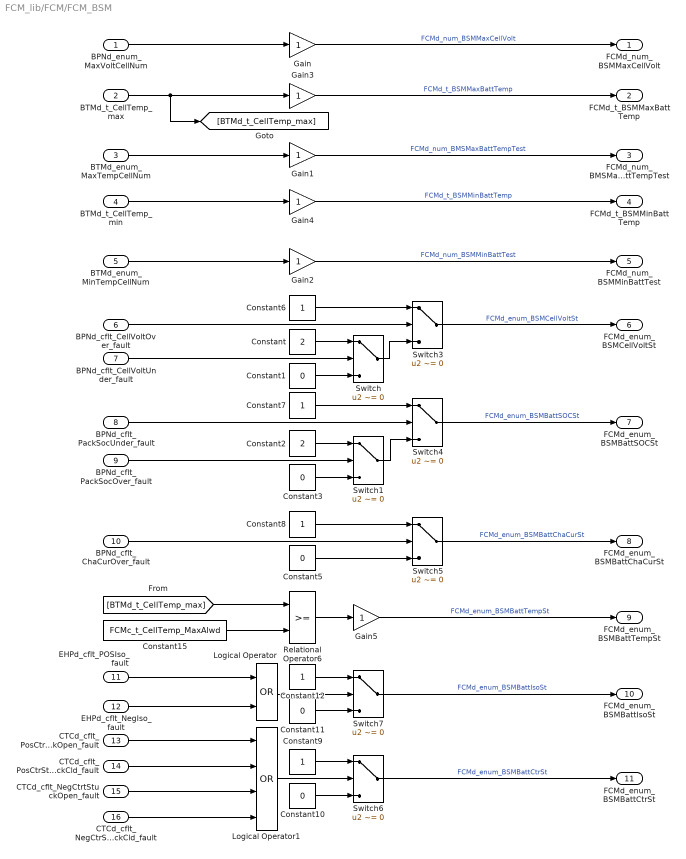
== system FCM_lib/FCM/FCM_BSM ==
  BPNd_enum_MaxVoltCellNum : Inport
  BTMd_t_CellTemp_max : Inport  Port=2
  BTMd_enum_MaxTempCellNum : Inport  Port=3
  BTMd_t_CellTemp_min : Inport  Port=4
  BTMd_enum_MinTempCellNum : Inport  Port=5
  BPNd_cflt_CellVoltOver_fault : Inport  Port=6
  BPNd_cflt_CellVoltUnder_fault : Inport  Port=7
  BPNd_cflt_PackSocUnder_fault : Inport  Port=8
  BPNd_cflt_PackSocOver_fault : Inport  Port=9
  BPNd_cflt_ChaCurOver_fault : Inport  Port=10
  EHPd_cflt_POSIso_fault : Inport  Port=11
  EHPd_cflt_NegIso_fault : Inport  Port=12
  CTCd_cflt_PosCtrStuckOpen_fault : Inport  Port=13
  CTCd_cflt_PosCtrStuckCld_fault : Inport  Port=14
  CTCd_cflt_NegCtrtStuckOpen_fault : Inport  Port=15
  CTCd_cflt_NegCtrStuckCld_fault : Inport  Port=16
  Constant : Constant  Value=2  OutDataTypeMode=uint8  OutDataTypeStr=uint8
  Constant{1,3,5,10..11} (5 alike) : Constant  Value=0  OutDataTypeMode=uint8  OutDataTypeStr=uint8
  Constant{6..9,12} (5 alike) : Constant  OutDataTypeMode=uint8  OutDataTypeStr=uint8
  Constant15 : Constant  Value=FCMc_t_CellTemp_MaxAlwd
  Constant2 : Constant  Value=2  OutDataTypeMode=uint8  OutDataTypeStr=uint8
  Gain{,1..5} (6 alike) : Gain  OutDataTypeStr=Inherit: Inherit via back propagation
  Logical Operator : Logic  Operator=OR  AllPortsSameDT=off  OutDataTypeMode=boolean  OutDataTypeStr=boolean
  Logical Operator1 : Logic  Operator=OR  Inputs=4  AllPortsSameDT=off  OutDataTypeMode=boolean  OutDataTypeStr=boolean
  Relational Operator6 : RelationalOperator  LogicOutDataTypeMode=boolean  OutDataTypeStr=boolean
  Switch : Switch  Criteria=u2 ~= 0
  Switch1 : Switch  Criteria=u2 ~= 0
  Switch{3..7} (5 alike) : Switch  Criteria=u2 ~= 0  OutDataTypeStr=Inherit: Inherit via back propagation
  FCMd_num_BSMMaxCellVolt : Outport
  FCMd_t_BSMMaxBattTemp : Outport  Port=2
  FCMd_num_BMSMaxBattTempTest : Outport  Port=3
  FCMd_t_BSMMinBattTemp : Outport  Port=4
  FCMd_num_BSMMinBattTest : Outport  Port=5
  FCMd_enum_BSMCellVoltSt : Outport  Port=6
  FCMd_enum_BSMBattSOCSt : Outport  Port=7
  FCMd_enum_BSMBattChaCurSt : Outport  Port=8
  FCMd_enum_BSMBattTempSt : Outport  Port=9
  FCMd_enum_BSMBattIsoSt : Outport  Port=10
  FCMd_enum_BSMBattCtrSt : Outport  Port=11
  wires:
  Constant15/1 -> Relational Operator6/2
  Gain5/1 -> FCMd_enum_BSMBattTempSt/1  "FCMd_enum_BSMBattTempSt"
  Relational Operator6/1 -> Gain5/1
  [BTMd_t_CellTemp_max] -> Relational Operator6/1
  Switch/1 -> Switch3/3
  Switch3/1 -> FCMd_enum_BSMCellVoltSt/1  "FCMd_enum_BSMCellVoltSt"
  Switch4/1 -> FCMd_enum_BSMBattSOCSt/1  "FCMd_enum_BSMBattSOCSt"
  Switch5/1 -> FCMd_enum_BSMBattChaCurSt/1  "FCMd_enum_BSMBattChaCurSt"
  BPNd_cflt_CellVoltOver_fault/1 -> Switch3/2
  BPNd_cflt_PackSocOver_fault/1 -> Switch1/2
  Switch1/1 -> Switch4/3
  BPNd_cflt_PackSocUnder_fault/1 -> Switch4/2
  Constant5/1 -> Switch5/3
  Switch7/1 -> FCMd_enum_BSMBattIsoSt/1  "FCMd_enum_BSMBattIsoSt"
  Switch6/1 -> FCMd_enum_BSMBattCtrSt/1  "FCMd_enum_BSMBattCtrSt"
  Logical Operator/1 -> Switch7/2
  BPNd_enum_MaxVoltCellNum/1 -> Gain/1
  Gain/1 -> FCMd_num_BSMMaxCellVolt/1  "FCMd_num_BSMMaxCellVolt"
  Gain3/1 -> FCMd_t_BSMMaxBattTemp/1  "FCMd_t_BSMMaxBattTemp"
  BTMd_t_CellTemp_max/1 -> Gain3/1, [BTMd_t_CellTemp_max]
  BTMd_enum_MaxTempCellNum/1 -> Gain1/1
  Gain4/1 -> FCMd_t_BSMMinBattTemp/1  "FCMd_t_BSMMinBattTemp"
  BTMd_t_CellTemp_min/1 -> Gain4/1
  BTMd_enum_MinTempCellNum/1 -> Gain2/1
  Logical Operator1/1 -> Switch6/2
  Gain1/1 -> FCMd_num_BMSMaxBattTempTest/1  "FCMd_num_BMSMaxBattTempTest"
  Gain2/1 -> FCMd_num_BSMMinBattTest/1  "FCMd_num_BSMMinBattTest"
  BPNd_cflt_CellVoltUnder_fault/1 -> Switch/2
  Constant/1 -> Switch/1
  Constant1/1 -> Switch/3
  Constant2/1 -> Switch1/1
  Constant3/1 -> Switch1/3
  Constant6/1 -> Switch3/1
  Constant7/1 -> Switch4/1
  Constant8/1 -> Switch5/1
  EHPd_cflt_POSIso_fault/1 -> Logical Operator/1
  EHPd_cflt_NegIso_fault/1 -> Logical Operator/2
  CTCd_cflt_PosCtrStuckOpen_fault/1 -> Logical Operator1/1
  CTCd_cflt_PosCtrStuckCld_fault/1 -> Logical Operator1/2
  CTCd_cflt_NegCtrtStuckOpen_fault/1 -> Logical Operator1/3
  CTCd_cflt_NegCtrStuckCld_fault/1 -> Logical Operator1/4
  Constant9/1 -> Switch6/1
  Constant10/1 -> Switch6/3
  Constant12/1 -> Switch7/1
  Constant11/1 -> Switch7/3
  BPNd_cflt_ChaCurOver_fault/1 -> Switch5/2

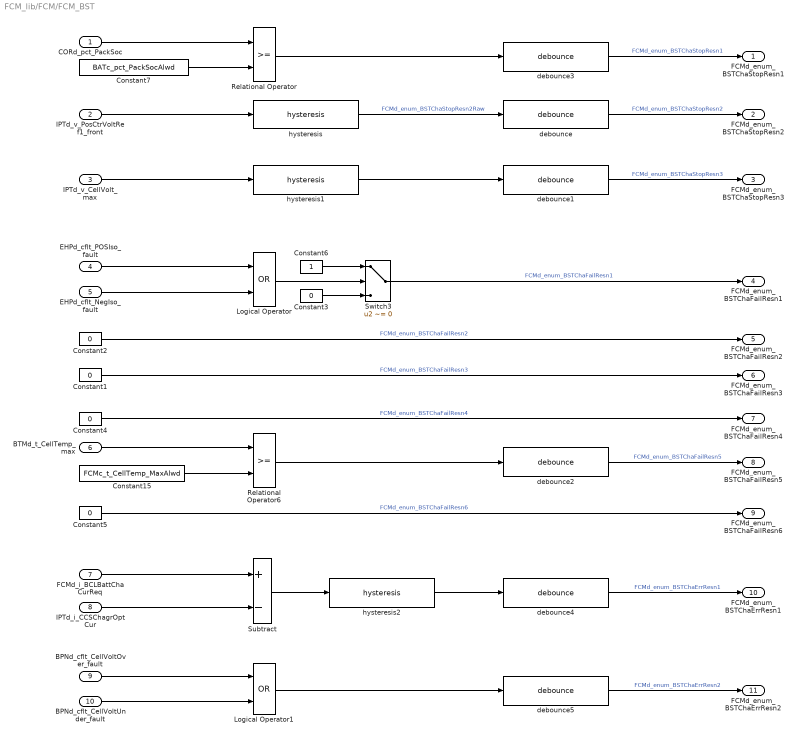
== system FCM_lib/FCM/FCM_BST ==
  CORd_pct_PackSoc : Inport
  IPTd_v_PosCtrVoltRef1_front : Inport  Port=2
  IPTd_v_CellVolt_max : Inport  Port=3
  EHPd_cflt_POSIso_fault : Inport  Port=4
  EHPd_cflt_NegIso_fault : Inport  Port=5
  BTMd_t_CellTemp_max : Inport  Port=6
  FCMd_i_BCLBattChaCurReq : Inport  Port=7
  IPTd_i_CCSChagrOptCur : Inport  Port=8
  BPNd_cflt_CellVoltOver_fault : Inport  Port=9
  BPNd_cflt_CellVoltUnder_fault : Inport  Port=10
  Constant{1..5} (5 alike) : Constant  Value=0  OutDataTypeMode=uint8  OutDataTypeStr=uint8
  Constant15 : Constant  Value=FCMc_t_CellTemp_MaxAlwd
  Constant6 : Constant  OutDataTypeMode=uint8  OutDataTypeStr=uint8
  Constant7 : Constant  Value=BATc_pct_PackSocAlwd
  Logical Operator : Logic  Operator=OR  AllPortsSameDT=off  OutDataTypeMode=boolean  OutDataTypeStr=boolean
  Logical Operator1 : Logic  Operator=OR  AllPortsSameDT=off  OutDataTypeMode=boolean  OutDataTypeStr=boolean
  Relational Operator : RelationalOperator  LogicOutDataTypeMode=boolean  LogicDataType=fixdt(0, 8)  OutDataTypeStr=boolean
  Relational Operator6 : RelationalOperator  LogicOutDataTypeMode=boolean  OutDataTypeStr=boolean
  Subtract : Sum  Inputs=+-
  Switch3 : Switch  Criteria=u2 ~= 0  OutDataTypeStr=Inherit: Inherit via back propagation
  debounce : Defined_Functionality/debounce  SystemSampleTime=-1  debounce_time=FCMc_tm_PackVoltDeb
      settings: AttributesFormatString=[DEBOUNCE_TIME=%<debounce_time>]
  debounce1 : Defined_Functionality/debounce  SystemSampleTime=-1  debounce_time=FCMc_tm_CellVoltDeb
      settings: AttributesFormatString=[DEBOUNCE_TIME=%<debounce_time>]
  debounce2 : Defined_Functionality/debounce  SystemSampleTime=-1  debounce_time=FCMc_tm_CellTempDeb
      settings: AttributesFormatString=[DEBOUNCE_TIME=%<debounce_time>]
  debounce3 : Defined_Functionality/debounce  SystemSampleTime=-1  debounce_time=FCMc_tm_PackSocDeb
      settings: AttributesFormatString=[DEBOUNCE_TIME=%<debounce_time>]
  debounce4 : Defined_Functionality/debounce  SystemSampleTime=-1  debounce_time=FCMc_tm_CurOverDeb
      settings: AttributesFormatString=[DEBOUNCE_TIME=%<debounce_time>]
  debounce5 : Defined_Functionality/debounce  SystemSampleTime=-1  debounce_time=FCMc_tm_CurOverDeb
      settings: AttributesFormatString=[DEBOUNCE_TIME=%<debounce_time>]
  hysteresis : Defined_Functionality/hysteresis  SystemSampleTime=-1  upper_limit=BATc_v_PackVoltChaAlwdUp  lower_limit=BATc_v_PackVoltChaAlwdDown
      settings: AttributesFormatString=[UPPER_LIMIT=%<upper_limit>]\n[LOWER_LIMIT=%<lower_limit>]
  hysteresis1 : Defined_Functionality/hysteresis  SystemSampleTime=-1  upper_limit=BATc_v_CellVolt_MaxAlwdUp  lower_limit=BATc_v_CellVolt_MaxAlwdDown
      settings: AttributesFormatString=[UPPER_LIMIT=%<upper_limit>]\n[LOWER_LIMIT=%<lower_limit>]
  hysteresis2 : Defined_Functionality/hysteresis  SystemSampleTime=-1  upper_limit=FCMc_i_ChagrCurOverDeltaUp  lower_limit=FCMc_i_ChagrCurOverDeltaDn
      settings: AttributesFormatString=[UPPER_LIMIT=%<upper_limit>]\n[LOWER_LIMIT=%<lower_limit>]
  FCMd_enum_BSTChaStopResn1 : Outport
  FCMd_enum_BSTChaStopResn2 : Outport  Port=2
  FCMd_enum_BSTChaStopResn3 : Outport  Port=3
  FCMd_enum_BSTChaFailResn1 : Outport  Port=4
  FCMd_enum_BSTChaFailResn2 : Outport  Port=5
  FCMd_enum_BSTChaFailResn3 : Outport  Port=6
  FCMd_enum_BSTChaFailResn4 : Outport  Port=7
  FCMd_enum_BSTChaFailResn5 : Outport  Port=8
  FCMd_enum_BSTChaFailResn6 : Outport  Port=9
  FCMd_enum_BSTChaErrResn1 : Outport  Port=10
  FCMd_enum_BSTChaErrResn2 : Outport  Port=11
  wires:
  debounce5/1 -> FCMd_enum_BSTChaErrResn2/1  "FCMd_enum_BSTChaErrResn2"
  debounce4/1 -> FCMd_enum_BSTChaErrResn1/1  "FCMd_enum_BSTChaErrResn1"
  debounce3/1 -> FCMd_enum_BSTChaStopResn1/1  "FCMd_enum_BSTChaStopResn1"
  debounce2/1 -> FCMd_enum_BSTChaFailResn5/1  "FCMd_enum_BSTChaFailResn5"
  debounce1/1 -> FCMd_enum_BSTChaStopResn3/1  "FCMd_enum_BSTChaStopResn3"
  debounce/1 -> FCMd_enum_BSTChaStopResn2/1  "FCMd_enum_BSTChaStopResn2"
  Subtract/1 -> hysteresis2/1
  Relational Operator6/1 -> debounce2/1
  BTMd_t_CellTemp_max/1 -> Relational Operator6/1
  Constant15/1 -> Relational Operator6/2
  Constant3/1 -> Switch3/3
  Constant6/1 -> Switch3/1
  Logical Operator/1 -> Switch3/2
  Switch3/1 -> FCMd_enum_BSTChaFailResn1/1  "FCMd_enum_BSTChaFailResn1"
  Constant7/1 -> Relational Operator/2
  CORd_pct_PackSoc/1 -> Relational Operator/1
  IPTd_v_PosCtrVoltRef1_front/1 -> hysteresis/1
  hysteresis/1 -> debounce/1  "FCMd_enum_BSTChaStopResn2Raw"
  hysteresis1/1 -> debounce1/1
  IPTd_v_CellVolt_max/1 -> hysteresis1/1
  EHPd_cflt_POSIso_fault/1 -> Logical Operator/1
  EHPd_cflt_NegIso_fault/1 -> Logical Operator/2
  hysteresis2/1 -> debounce4/1
  Logical Operator1/1 -> debounce5/1
  Constant2/1 -> FCMd_enum_BSTChaFailResn2/1  "FCMd_enum_BSTChaFailResn2"
  Constant1/1 -> FCMd_enum_BSTChaFailResn3/1  "FCMd_enum_BSTChaFailResn3"
  Constant4/1 -> FCMd_enum_BSTChaFailResn4/1  "FCMd_enum_BSTChaFailResn4"
  Constant5/1 -> FCMd_enum_BSTChaFailResn6/1  "FCMd_enum_BSTChaFailResn6"
  Relational Operator/1 -> debounce3/1
  BPNd_cflt_CellVoltOver_fault/1 -> Logical Operator1/1
  BPNd_cflt_CellVoltUnder_fault/1 -> Logical Operator1/2
  FCMd_i_BCLBattChaCurReq/1 -> Subtract/1
  IPTd_i_CCSChagrOptCur/1 -> Subtract/2

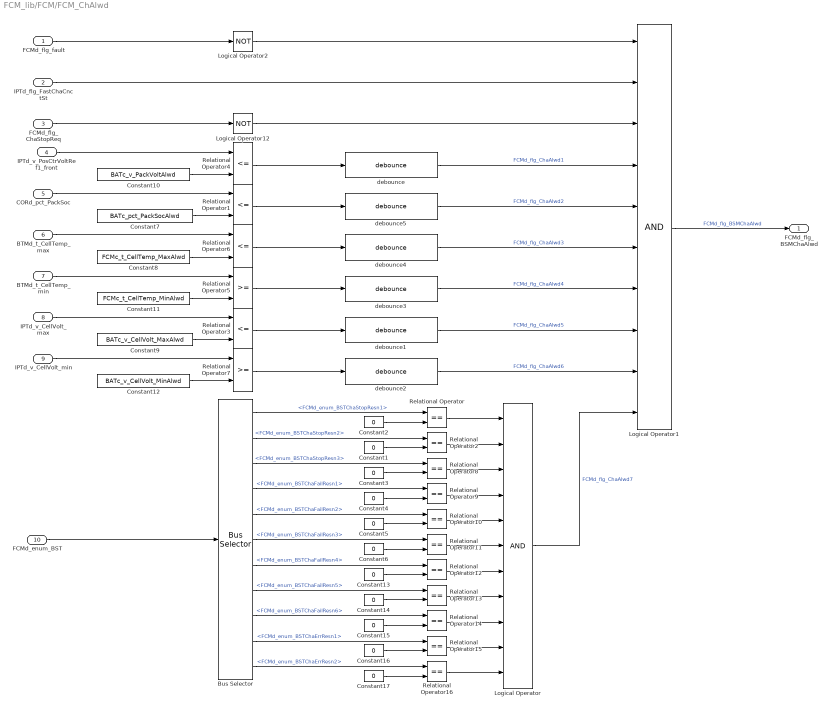
== system FCM_lib/FCM/FCM_ChAlwd ==
  FCMd_flg_fault : Inport
  IPTd_flg_FastChaCnctSt : Inport  Port=2
  FCMd_flg_ChaStopReq : Inport  Port=3
  IPTd_v_PosCtrVoltRef1_front : Inport  Port=4
  CORd_pct_PackSoc : Inport  Port=5
  BTMd_t_CellTemp_max : Inport  Port=6
  BTMd_t_CellTemp_min : Inport  Port=7
  IPTd_v_CellVolt_max : Inport  Port=8
  IPTd_v_CellVolt_min : Inport  Port=9
  FCMd_enum_BST : Inport  Port=10
  Bus Selector : BusSelector  OutputSignals=FCMd_enum_BSTChaStopResn1,FCMd_enum_BSTChaStopResn2,FCMd_enum_BSTChaStopResn3,FCMd_enum_BSTChaFailResn1,FCMd_enum_BSTChaFailResn2,FCMd_enum_BSTChaFailResn3,FCMd_enum_BSTChaFailResn4,FCMd_enum_BSTChaFailResn5,FCMd_enum_BSTChaFailResn6,FCMd_enum_BSTChaErrResn1,FCMd_enum_BSTChaErrResn2
  Constant{1..6,13..17} (11 alike) : Constant  Value=0  OutDataTypeMode=uint8  OutDataTypeStr=uint8
  Constant10 : Constant  Value=BATc_v_PackVoltAlwd
  Constant11 : Constant  Value=FCMc_t_CellTemp_MinAlwd
  Constant12 : Constant  Value=BATc_v_CellVolt_MinAlwd
  Constant7 : Constant  Value=BATc_pct_PackSocAlwd
  Constant8 : Constant  Value=FCMc_t_CellTemp_MaxAlwd
  Constant9 : Constant  Value=BATc_v_CellVolt_MaxAlwd
  Logical Operator : Logic  Inputs=11  AllPortsSameDT=off
  Logical Operator1 : Logic  Inputs=10  AllPortsSameDT=off  OutDataTypeMode=boolean  OutDataTypeStr=boolean
  Logical Operator12 : Logic  Operator=NOT  Inputs=1  AllPortsSameDT=off  OutDataTypeMode=boolean  OutDataTypeStr=boolean
  Logical Operator2 : Logic  Operator=NOT  Inputs=1  AllPortsSameDT=off  OutDataTypeMode=boolean  OutDataTypeStr=boolean
  Relational Operator{,2,8..16} (11 alike) : RelationalOperator  Operator===  LogicOutDataTypeMode=boolean  LogicDataType=fixdt(0, 8)  OutDataTypeStr=boolean
  Relational Operator{1,3..4,6} (4 alike) : RelationalOperator  Operator=<=  LogicOutDataTypeMode=boolean  OutDataTypeStr=boolean
  Relational Operator5 : RelationalOperator  LogicOutDataTypeMode=boolean  OutDataTypeStr=boolean
  Relational Operator7 : RelationalOperator  LogicOutDataTypeMode=boolean  OutDataTypeStr=boolean
  debounce : Defined_Functionality/debounce  SystemSampleTime=-1  debounce_time=FCMc_tm_PackVoltDeb
      settings: AttributesFormatString=[DEBOUNCE_TIME=%<debounce_time>]
  debounce{1..5} (5 alike) : Defined_Functionality/debounce  SystemSampleTime=-1  debounce_time=FCMc_tm_CellVoltDeb
      settings: AttributesFormatString=[DEBOUNCE_TIME=%<debounce_time>]
  FCMd_flg_BSMChaAlwd : Outport
  wires:
  Relational Operator1/1 -> debounce5/1
  debounce5/1 -> Logical Operator1/5  "FCMd_flg_ChaAlwd2"
  debounce4/1 -> Logical Operator1/6  "FCMd_flg_ChaAlwd3"
  debounce3/1 -> Logical Operator1/7  "FCMd_flg_ChaAlwd4"
  debounce2/1 -> Logical Operator1/9  "FCMd_flg_ChaAlwd6"
  debounce1/1 -> Logical Operator1/8  "FCMd_flg_ChaAlwd5"
  debounce/1 -> Logical Operator1/4  "FCMd_flg_ChaAlwd1"
  Logical Operator/1 -> Logical Operator1/10  "FCMd_flg_ChaAlwd7"
  Relational Operator16/1 -> Logical Operator/11
  Relational Operator15/1 -> Logical Operator/10
  Relational Operator14/1 -> Logical Operator/9
  Relational Operator13/1 -> Logical Operator/8
  Relational Operator12/1 -> Logical Operator/7
  Relational Operator11/1 -> Logical Operator/6
  Relational Operator10/1 -> Logical Operator/5
  Relational Operator9/1 -> Logical Operator/4
  Relational Operator8/1 -> Logical Operator/3
  Relational Operator2/1 -> Logical Operator/2
  Constant17/1 -> Relational Operator16/2
  Constant16/1 -> Relational Operator15/2
  Constant15/1 -> Relational Operator14/2
  Constant14/1 -> Relational Operator13/2
  Constant13/1 -> Relational Operator12/2
  Constant6/1 -> Relational Operator11/2
  Bus Selector/11 -> Relational Operator16/1  "<FCMd_enum_BSTChaErrResn2>"
  Bus Selector/10 -> Relational Operator15/1  "<FCMd_enum_BSTChaErrResn1>"
  Bus Selector/9 -> Relational Operator14/1  "<FCMd_enum_BSTChaFailResn6>"
  Bus Selector/8 -> Relational Operator13/1  "<FCMd_enum_BSTChaFailResn5>"
  Bus Selector/7 -> Relational Operator12/1  "<FCMd_enum_BSTChaFailResn4>"
  Bus Selector/6 -> Relational Operator11/1  "<FCMd_enum_BSTChaFailResn3>"
  Constant5/1 -> Relational Operator10/2
  Bus Selector/5 -> Relational Operator10/1  "<FCMd_enum_BSTChaFailResn2>"
  Constant4/1 -> Relational Operator9/2
  Bus Selector/4 -> Relational Operator9/1  "<FCMd_enum_BSTChaFailResn1>"
  Constant3/1 -> Relational Operator8/2
  Bus Selector/3 -> Relational Operator8/1  "<FCMd_enum_BSTChaStopResn3>"
  Bus Selector/2 -> Relational Operator2/1  "<FCMd_enum_BSTChaStopResn2>"
  Constant1/1 -> Relational Operator2/2
  Relational Operator/1 -> Logical Operator/1
  Bus Selector/1 -> Relational Operator/1  "<FCMd_enum_BSTChaStopResn1>"
  Constant2/1 -> Relational Operator/2
  FCMd_enum_BST/1 -> Bus Selector/1
  Logical Operator1/1 -> FCMd_flg_BSMChaAlwd/1  "FCMd_flg_BSMChaAlwd"
  Relational Operator7/1 -> debounce2/1
  Relational Operator3/1 -> debounce1/1
  IPTd_flg_FastChaCnctSt/1 -> Logical Operator1/2
  CORd_pct_PackSoc/1 -> Relational Operator1/1
  Constant7/1 -> Relational Operator1/2
  IPTd_v_CellVolt_max/1 -> Relational Operator3/1
  Constant9/1 -> Relational Operator3/2
  Constant10/1 -> Relational Operator4/2
  IPTd_v_PosCtrVoltRef1_front/1 -> Relational Operator4/1
  Constant11/1 -> Relational Operator5/2
  BTMd_t_CellTemp_min/1 -> Relational Operator5/1
  Constant8/1 -> Relational Operator6/2
  BTMd_t_CellTemp_max/1 -> Relational Operator6/1
  FCMd_flg_fault/1 -> Logical Operator2/1
  IPTd_v_CellVolt_min/1 -> Relational Operator7/1
  Constant12/1 -> Relational Operator7/2
  FCMd_flg_ChaStopReq/1 -> Logical Operator12/1
  Logical Operator2/1 -> Logical Operator1/1
  Logical Operator12/1 -> Logical Operator1/3
  Relational Operator4/1 -> debounce/1
  Relational Operator6/1 -> debounce4/1
  Relational Operator5/1 -> debounce3/1

== system FCM_lib/FCM/FCM_fault ==
  FCMd_cflt_ChaCurDifOver_fault : Inport  OutDataType=fixdt(1, 16)  OutScaling=2^0
  FCMd_cflt_ChaVoltDifOver_fault : Inport  Port=2  OutDataType=fixdt(1, 16)  OutScaling=2^0
  Enable : EnablePort
  Logical Operator : Logic  Operator=OR  AllPortsSameDT=off  OutDataTypeMode=boolean  LogicDataType=fixdt(0, 8)  OutDataTypeStr=boolean
  FCMd_flg_fault : Outport  InitialOutput=[0]
  wires:
  Logical Operator/1 -> FCMd_flg_fault/1  "FCMd_flg_fault"
  FCMd_cflt_ChaCurDifOver_fault/1 -> Logical Operator/1
  FCMd_cflt_ChaVoltDifOver_fault/1 -> Logical Operator/2

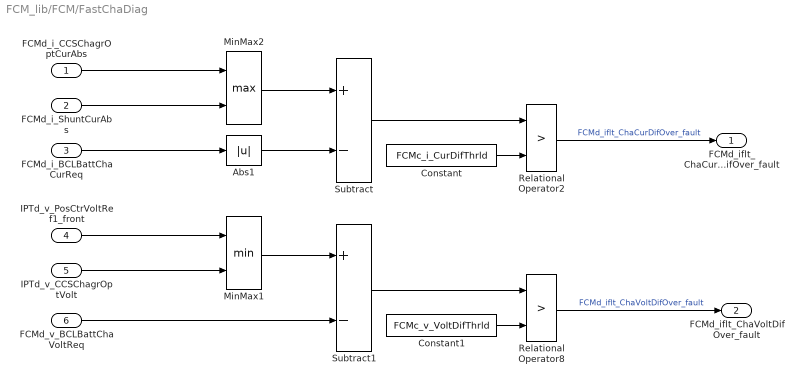
== system FCM_lib/FCM/FastChaDiag ==
  FCMd_i_CCSChagrOptCurAbs : Inport
  FCMd_i_ShuntCurAbs : Inport  Port=2
  FCMd_i_BCLBattChaCurReq : Inport  Port=3
  IPTd_v_PosCtrVoltRef1_front : Inport  Port=4  OutDataType=fixdt(1, 16)  OutScaling=2^0
  IPTd_v_CCSChagrOptVolt : Inport  Port=5
  FCMd_v_BCLBattChaVoltReq : Inport  Port=6
  Abs1 : Abs
  Constant : Constant  Value=FCMc_i_CurDifThrld
  Constant1 : Constant  Value=FCMc_v_VoltDifThrld
  MinMax1 : MinMax  Inputs=2  OutDataType=fixdt(1, 16)  OutScaling=2^0
  MinMax2 : MinMax  Function=max  Inputs=2  OutDataType=fixdt(1, 16)  OutScaling=2^0
  Relational Operator2 : RelationalOperator  Operator=>  LogicOutDataTypeMode=boolean  OutDataTypeStr=boolean
  Relational Operator8 : RelationalOperator  Operator=>  LogicOutDataTypeMode=boolean  OutDataTypeStr=boolean
  Subtract : Sum  Inputs=+-
  Subtract1 : Sum  Inputs=+-
  FCMd_iflt_ChaCurDifOver_fault : Outport  OutDataType=fixdt(1, 16)  OutScaling=2^0
  FCMd_iflt_ChaVoltDifOver_fault : Outport  Port=2  OutDataType=fixdt(1, 16)  OutScaling=2^0
  wires:
  MinMax2/1 -> Subtract/1
  Abs1/1 -> Subtract/2
  FCMd_i_ShuntCurAbs/1 -> MinMax2/2
  FCMd_i_CCSChagrOptCurAbs/1 -> MinMax2/1
  MinMax1/1 -> Subtract1/1
  IPTd_v_PosCtrVoltRef1_front/1 -> MinMax1/1
  FCMd_v_BCLBattChaVoltReq/1 -> Subtract1/2
  IPTd_v_CCSChagrOptVolt/1 -> MinMax1/2
  Subtract1/1 -> Relational Operator8/1
  Constant/1 -> Relational Operator2/2
  Subtract/1 -> Relational Operator2/1
  FCMd_i_BCLBattChaCurReq/1 -> Abs1/1
  Constant1/1 -> Relational Operator8/2
  Relational Operator2/1 -> FCMd_iflt_ChaCurDifOver_fault/1  "FCMd_iflt_ChaCurDifOver_fault"
  Relational Operator8/1 -> FCMd_iflt_ChaVoltDifOver_fault/1  "FCMd_iflt_ChaVoltDifOver_fault"

== system FCM_lib/FCM/FCM_BCL/debounce1 ==
  in : Inport  OutDataType=sfix(16)  OutScaling=2^0
  debounce : Stateflow chart  TreatAsAtomicUnit=on
  out : Outport  OutDataType=sfix(16)  OutScaling=2^0
  wires:
  debounce/1(out) -> out/1
  in/1 -> debounce/1(in)
